simulink model "MPC"  (R2020a)
settings: Solver=ode4  StartTime=0.0  StopTime=tend  FixedStep=1  RelTol=1e-3
InitFcn:
  | SetupParameters
StopFcn:
  | PlotResults
values from neighbouring files (symbols this model uses):
  A_KF = Abar * (I-M*Cbar)    [SetupParameters.m]
  alpha = 0.3    [SetupParameters.m]
  B_KF = [Bbar, Abar*M]    [SetupParameters.m]
  C_KF = eye(16)    [SetupParameters.m]
  Cbar = [plantD.C, zeros(q,p)]    [SetupParameters.m]
  D_KF = zeros(16,6)    [SetupParameters.m]
  I = eye(n+p)    [SetupParameters.m]
  Ts = 1    [SetupParameters.m]    (also in TestMPC.m; mpc_s_L2.m = block.DialogPrm(8).Data)
undefined symbols (not defined in the file or in its folder): M
libraries: cstblocks x1, simulink x1
settings Model: Creator=Charl  LastModifiedBy=Charl

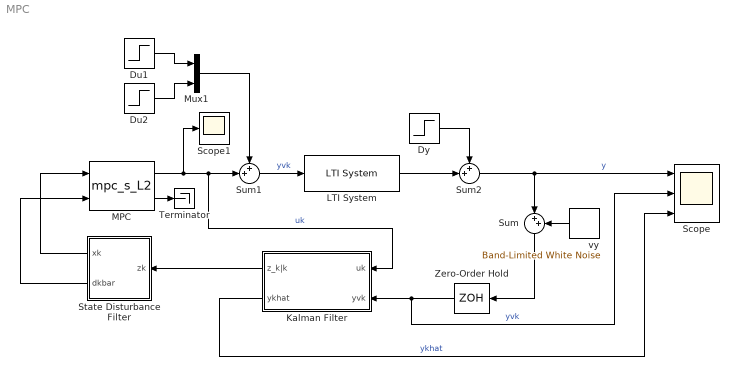
== system MPC ==
  Du1 : Step  Time=10  SampleTime=0
  Du2 : Step  Time=20  After=-1  SampleTime=0
  Dy : Step  Time=80  After=[1; -1]  SampleTime=0
  Kalman Filter : Subsystem
      settings: PortSchema="{\"entries\":[{\"content\":{\"sides\":[{\"content\":{\"connectorIds\":[\"Out1\",\"Out2\"]},\"type\":\"ConnectorPlacement.EquallySpacedRectSide\",\"uuid\":\"3cd62786-1984-41d0-8056-3af756c1ac1f\"},{\"content\":{\"connectorIds\":[\"In1\",\"In2\"],\"side\":\"RIGHT\"},\"type\":\"ConnectorPlacement.EquallySpacedRectSide\",\"uuid\":\"bfb72803-0fd3-4bc2-8890-c24e16713331\"},{\"content\":{\"connectorIds\":[],\"side\":\"TOP\"},\"type\":\"ConnectorPlacement.EquallySpacedRectSide\",\"uuid\":\"8d76b870-fa9c-4775-8c38-f291a42b27fa\"}]},\"type\":\"ConnectorPlacement.EquallySpacedConnector\",\"uuid\":\"fe1c535d-ee3a-4357-b747-4ea412b9dcf1\"}],\"packageUris\":[\"http://schema.mathworks.com/mf0/Connector/19700101\"],\"version\":\"1.0\"}"
  LTI System : cstblocks/LTI System  sys=Gp  IC=[]
  MPC : M-S-Function  FunctionName=mpc_s_L2  Parameters=Gd, YspArr, Np, Nb, Nc, Q, R, Ts
  Mux1 : Mux  Inputs=2
  Scope : Scope  NumInputPorts=3
  Scope1 : Scope
  State Disturbance Filter : Subsystem
      settings: PortSchema="{\"entries\":[{\"content\":{\"sides\":[{\"content\":{\"connectorIds\":[\"Out1\",\"Out2\"]},\"type\":\"ConnectorPlacement.EquallySpacedRectSide\",\"uuid\":\"063c4a96-47a1-4ba5-b380-f2535e65689f\"},{\"content\":{\"connectorIds\":[\"In1\"],\"side\":\"RIGHT\"},\"type\":\"ConnectorPlacement.EquallySpacedRectSide\",\"uuid\":\"12490f34-1dc5-4285-a463-ea026b076ed1\"},{\"content\":{\"connectorIds\":[],\"side\":\"TOP\"},\"type\":\"ConnectorPlacement.EquallySpacedRectSide\",\"uuid\":\"7aff2aed-48cc-43a1-bb93-aeccf421ef28\"}]},\"type\":\"ConnectorPlacement.EquallySpacedConnector\",\"uuid\":\"5a6b5c7e-4ce6-4bfe-ad60-0a1a27b03ee8\"}],\"packageUris\":[\"http://schema.mathworks.com/mf0/Connector/19700101\"],\"version\":\"1.0\"}"
  Sum : Sum  Inputs=|++
  Sum1 : Sum  Inputs=++|
  Sum2 : Sum  Inputs=++|
  Terminator : Terminator
  Zero-Order Hold : ZeroOrderHold  SampleTime=-1
  vy : simulink/Sources/Band-Limited White Noise  Cov=[0.1; 0.1]  Ts=Ts  seed=[3341]
  wires:
  MPC/1 -> Sum1/2, Kalman Filter/1(uk), Scope1/1  "uk"
  MPC/2 -> Terminator/1
  Sum2/1 -> Sum/1, Scope/1  "y"
  Sum1/1 -> LTI System/1  "yvk"
  Du1/1 -> Mux1/1
  Du2/1 -> Mux1/2
  Mux1/1 -> Sum1/1
  Kalman Filter/1(z_k|k) -> State Disturbance Filter/1(zk)
  State Disturbance Filter/1(xk) -> MPC/1
  State Disturbance Filter/2(dkbar) -> MPC/2
  Sum/1 -> Zero-Order Hold/1
  Dy/1 -> Sum2/1
  Zero-Order Hold/1 -> Scope/2, Kalman Filter/2(yvk)  "yvk"
  vy/1 -> Sum/2
  LTI System/1 -> Sum2/2
  Kalman Filter/2(ykhat) -> Scope/3  "ykhat"

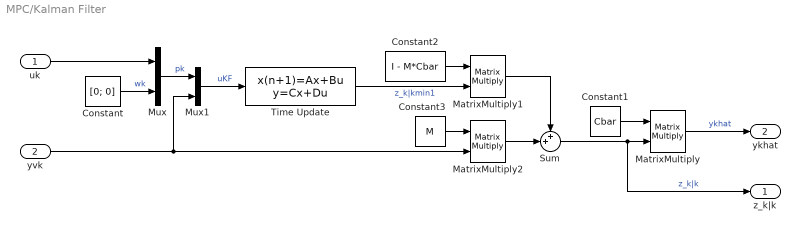
== system MPC/Kalman Filter ==
  uk : Inport
  yvk : Inport  Port=2
  Constant : Constant  Value=[0; 0]  SampleTime=Ts
  Constant1 : Constant  Value=Cbar
  Constant2 : Constant  Value=I - M*Cbar
  Constant3 : Constant  Value=M
  MatrixMultiply : Product  Multiplication=Matrix(*)
  MatrixMultiply1 : Product  Multiplication=Matrix(*)
  MatrixMultiply2 : Product  Multiplication=Matrix(*)
  Mux : Mux  Inputs=2
  Mux1 : Mux  Inputs=2
  Sum : Sum  Inputs=++|
  Time Update : DiscreteStateSpace  A=A_KF  B=B_KF  C=C_KF  D=D_KF  SampleTime=Ts
  z_k|k : Outport
  ykhat : Outport  Port=2
  wires:
  Mux/1 -> Mux1/1  "pk"
  MatrixMultiply1/1 -> Sum/1
  Mux1/1 -> Time Update/1  "uKF"
  Constant/1 -> Mux/2  "wk"
  Sum/1 -> z_k|k/1, MatrixMultiply/2  "z_k|k"
  MatrixMultiply2/1 -> Sum/2
  Time Update/1 -> MatrixMultiply1/2  "z_k|kmin1"
  Constant1/1 -> MatrixMultiply/1
  yvk/1 -> Mux1/2, MatrixMultiply2/2
  Constant2/1 -> MatrixMultiply1/1
  Constant3/1 -> MatrixMultiply2/1
  uk/1 -> Mux/1
  MatrixMultiply/1 -> ykhat/1  "ykhat"

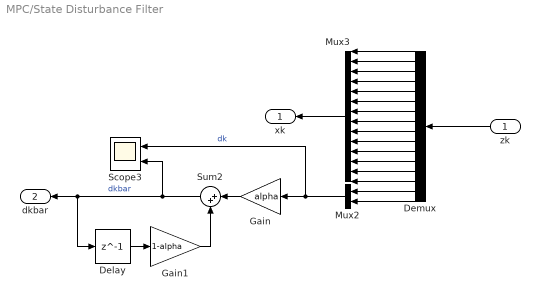
== system MPC/State Disturbance Filter ==
  zk : Inport
  Delay : Delay  DelayLength=1
  Demux : Demux  Outputs=16
  Gain : Gain  Gain=alpha
  Gain1 : Gain  Gain=1-alpha
  Mux2 : Mux  Inputs=2
  Mux3 : Mux  Inputs=14
  Scope3 : Scope  NumInputPorts=2
  Sum2 : Sum  Inputs=|++
  xk : Outport
  dkbar : Outport  Port=2
  wires:
  Gain/1 -> Sum2/1
  Mux2/1 -> Gain/1, Scope3/1  "dk"
  Sum2/1 -> dkbar/1, Delay/1, Scope3/2  "dkbar"
  Delay/1 -> Gain1/1
  Demux/12 -> Mux3/12
  Demux/16 -> Mux2/2
  Gain1/1 -> Sum2/2
  Mux3/1 -> xk/1
  Demux/6 -> Mux3/6
  Demux/3 -> Mux3/3
  zk/1 -> Demux/1
  Demux/8 -> Mux3/8
  Demux/7 -> Mux3/7
  Demux/15 -> Mux2/1
  Demux/13 -> Mux3/13
  Demux/1 -> Mux3/1
  Demux/9 -> Mux3/9
  Demux/5 -> Mux3/5
  Demux/4 -> Mux3/4
  Demux/14 -> Mux3/14
  Demux/10 -> Mux3/10
  Demux/2 -> Mux3/2
  Demux/11 -> Mux3/11
